simulink library "MotoLibrary"  (R2019b)
settings: Solver=VariableStepAuto  StartTime=0.0  StopTime=10.0  RelTol=1e-3
undefined symbols (not defined in the file or in its folder): Percentage
libraries: arduinolib x9, simulink x2, $bdroot x2
settings Model: Creator=JB  LastModifiedBy=JB

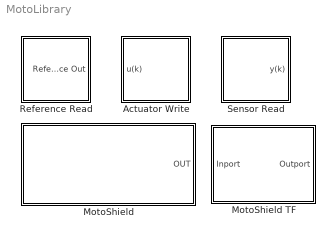
== system MotoLibrary ==
  Actuator Write : Subsystem  mask{inputType=Percentage (%), dir=Clockwise}
      mask prompts: inputType "Selected Input Type:"; dir "Spin Direction:"
      mask init:
      | if dir == 1
      |     direction = 1
      | else
      |     direction = 0
      | end
      mask TypeOptions inputType: Percentage (%) | Voltage (V) | PWM (8-bit)
      mask Callback inputType:
      | obj = get_param(gcb,'MaskObject');
      | txt = obj.getDialogControl('text');
      | input = get_param(gcb,'inputType');
      | if strcmp(input, 'Percentage (%)')
      |     txt.Prompt = 'Expected input value ranges between 0 - 100 %';
      | end
      | if strcmp(input, 'Voltage (V)')
      |     txt.Prompt = 'Expected input value ranges between 0 - 5 V';
      | end
      | if strcmp(input, 'PWM (8-bit)')
      |     txt.Prompt = 'Expected input value ranges between 0 - 255';
      | end
      mask TypeOptions dir: Clockwise | Counter-clockwise
      mask DialogControl DescGroupVar Prompt: MotoShield Actuator
      mask DialogControl DescTextVar Prompt: This block writes PWM signal to motor in MotoShield device. Expected input value varies based on the Selected Input Type.
      mask DialogControl text Prompt: Expected input value ranges between 0 - 100 %
      mask Display: image('assets\MotoShield_Motor.svg');
  MotoShield : Subsystem  mask{inputType=Internal Reference, direction=Clockwise, calibration=Perform calibration, manualLower=1010, manualUpper=2120, Ts=0.1}
      mask prompts: inputType "Form of input:"; calibration "Calibration values:"; manualLower "Minimal value:"; manualUpper "Maximal value:"; Ts "Sampling time (s):"
      mask init:
      | set_param(gcb, 'MaskSelfModifiable', 'on');
      | if inputType == 1
      |     if getSimulinkBlockHandle([gcb '/Inport']) == -1
      |         delete_line(gcb,'Reference Read/1','Saturation/1');
      |         add_block('built-in/Inport',[gcb '/Inport']);
      |         add_line(gcb,'Inport/1','Saturation/1');
      |     end
      | elseif inputType == 2
      |     if getSimulinkBlockHandle([gcb '/Inport']) > 0
      |         delete_line(gcb,'Inport/1','Saturation/1');
      |         delete_block([gcb '/Inport']);
      |         add_line(gcb,'Reference Read/1','Saturation/1');
      |     end
      | end
      mask TypeOptions inputType: External Reference | Internal Reference
      mask TypeOptions direction: Clockwise | Counterclockwise
      mask TypeOptions calibration: Perform calibration | Use default values | Set values manually
      mask Callback calibration:
      | currentBlock = gcb
      | in = get_param(currentBlock,'calibration');
      | menu = Simulink.Mask.get(currentBlock);
      | txt = menu.getDialogControl('calText');
      | lower = menu.getParameter('manualLower');
      | upper = menu.getParameter('manualUpper');
      | if strcmp(in,'Perform calibration')
      | lower.Enabled='off';
      | lower.Visible='off';
      | upper.Enabled='off';
      | upper.Visible='off';
      | txt.Visible='off';
      | elseif strcmp(in,'Use default values')
      | lower.Enabled='off';
      | lower.Visible='on';
      | upper.Enabled='off';
      | upper.Visible='on';
      | set_param(gcb,'manualLower',num2str(800));
      | set_param(gcb,'manualUpper',num2str(2050));
      | elseif strcmp(in,'Set values manually')
      | lower.Enabled='on';
      | lower.Visible='on';
      | upper.Enabled='on';
      | upper.Visible='on';
      | txt.Visible='on';
      | end
      mask DialogControl DescGroupVar Prompt: MotoShield
      mask DialogControl DescTextVar Prompt: This blocks writes actuator value and measures the angular velocity of the Motor. The reference value can be chosen either as an external signal or internal potentiometers value.  Since the output signal is expressed in percentages, calibration values have to be either specified or aquired via calibration. It is recommended to perform a calibration for accurate percentage formatting.
      mask DialogControl Control2 Prompt: Notice: Calibration is applicable only for unladen state.
      mask DialogControl calText Prompt: Calibration values ought to be entered as angular velocity in number of impulses per sample.
      mask Display: image('assets\MotoShield.svg');
  MotoShield TF : Subsystem  mask{inputType=Percentage (%), outputType=Rotations per minute (RPM), maxValue=0, minValue=0}
      mask prompts: inputType "Input value type:"; outputType "Output value type:"; maxValue "Calibration maximum value:"; minValue "Calibration minimum value:"
      mask TypeOptions inputType: Percentage (%) | RMS Voltage (V)
      mask TypeOptions outputType: Rotations per minute (RPM) | Radians per second (rad/s) | Percentage (%)
      mask Callback outputType:
      | CurrentBlock = gcb;
      | cal = get_param(CurrentBlock,'outputType');
      | menu = Simulink.Mask.get(CurrentBlock);
      | txt = menu.getDialogControl('calText');
      | min = menu.getParameter('minValue');
      | max = menu.getParameter('maxValue');
      | if strcmp(cal,'Percentage (%)')
      | min.Enabled='on';
      | min.Visible='on';
      | max.Enabled='on';
      | max.Visible='on';
      | txt.Visible='on';
      | set_param(gcb,'minValue',num2str(488));
      | set_param(gcb,'maxValue',num2str(976));
      | else
      | min.Enabled='off';
      | min.Visible='off';
      | max.Enabled='off';
      | max.Visible='off';
      | txt.Visible='off';
      | end
      mask DialogControl DescGroupVar Prompt: OptoShield TF
      mask DialogControl DescTextVar Prompt: The block represents the simplified second-order continuous transfer function of the MotoShield device.   Both input and output are availible in several value types. If output type selected is Percentage (%), calibration values are required. The calibration values have to be stated in radians per second.
      mask DialogControl Container2 Prompt: Parameters
      mask DialogControl calText Prompt: Calibration values are supposed to represent output range of the Motor in Radian per second (rad/s).
      mask Display: image('assets\MotoShield_TF.svg');
  Reference Read : Subsystem  mask{radio=Percentage (%), Ts=0.1}
      mask prompts: radio "Readout Type"; Ts "Sample time (s):"
      mask init:
      | if radio==1 
      | gainValue = (100/1023);       
      | end
      | if radio==2
      | gainValue = (5/1023);
      | end
      | if radio==3
      | gainValue = 1;             
      | end
      mask TypeOptions radio: Percentage (%) | Voltage (V) | Analog value (10-bit ADC)
      mask DialogControl DescGroupVar Prompt: MotoShield Potentiometer
      mask DialogControl DescTextVar Prompt: This blocks reads potentiometer wiper value on the MotoShield device. Multiple output value types availible.
      mask Display: image('assets\Potentiometer.svg');
  Sensor Read : Subsystem  mask{outputType=Percentage (%), calibrationValues=Use default values, minValue=800, maxValue=2060, Ts=0.1}
      mask prompts: outputType "Selected Output Type:"; calibrationValues "Calibration Values:"; minValue "Minimal Value:"; maxValue "Maximal Value:"; Ts "Sample time (s):"
      mask TypeOptions outputType: Percentage (%) | Rotation per minute (RPM) | Radian per second (rad/s)
      mask Callback outputType:
      | CurrentBlock = gcb;
      | out = get_param(CurrentBlock,'outputType');
      | menu = Simulink.Mask.get(CurrentBlock);
      | txt = menu.getDialogControl('calText');
      | calopt = menu.getParameter('calibrationValues');
      | min = menu.getParameter('minValue');
      | max = menu.getParameter('maxValue');
      | if strcmp(out,'Percentage (%)')
      | calopt.Enabled='on';
      | calopt.Visible='on';
      | txt.Visible='on';
      | else
      | calopt.Enabled='off';
      | calopt.Visible='off';
      | min.Visible = 'off'
      | max.Visible = 'off'
      | txt.Visible='off';
      | end
      mask TypeOptions calibrationValues: Set values manually | Use default values
      mask Callback calibrationValues:
      | CurrentBlock = gcbh;
      | cal = get_param(CurrentBlock,'calibrationValues');
      | menu = Simulink.Mask.get(CurrentBlock);
      | min = menu.getParameter('minValue');
      | max = menu.getParameter('maxValue');
      | if strcmp(cal,'Set values manually')
      | min.Enabled='on';
      | min.Visible='on';
      | max.Enabled='on';
      | max.Visible='on';
      | elseif strcmp(cal,'Use default values')
      | set_param(gcb,'minValue',num2str(800));
      | set_param(gcb,'maxValue',num2str(2060));
      | min.Enabled='off';
      | min.Visible='on';
      | max.Enabled='off';
      | max.Visible='on';
      | end
      mask DialogControl DescGroupVar Prompt: Hall Sensor
      mask DialogControl DescTextVar Prompt: This block outputs the angular velocity of the Motor. Multiple output value types available.
      mask DialogControl calText Prompt: Calibration values ought to be entered as angular velocity in number of impulses per sample.
      mask Display: image('assets\MotoShield_Sensor.svg');

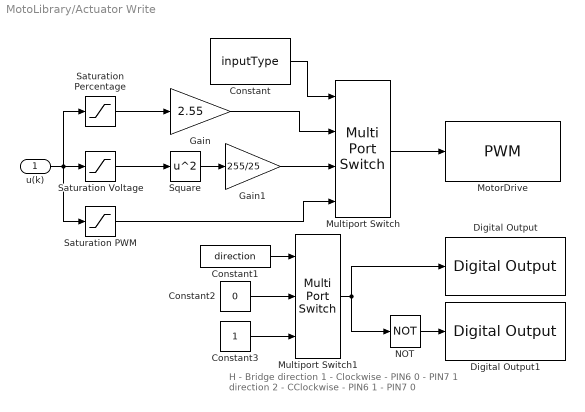
== system MotoLibrary/Actuator Write ==
  note: H - Bridge
      | direction 1 - Clockwise - PIN6 0 - PIN7 1
      | direction 2 - CClockwise - PIN6 1 - PIN7 0
  u(k) : Inport
  Constant : Constant  Value=inputType
  Constant1 : Constant  Value=direction
  Constant2 : Constant  Value=0
  Constant3 : Constant
  Digital Output : arduinolib/Digital Output  pinNumber=6  blockPlatform=arduino
  Digital Output1 : arduinolib/Digital Output  pinNumber=7  blockPlatform=arduino
  Gain : Gain  Gain=2.55
  Gain1 : Gain  Gain=255/25
  MotorDrive : arduinolib/PWM  pinNumber=5  EnableInputFrequency=off  InitialFrequency=2000  InitialDutyCycle=0  NotificationType=None  blockPlatform=arduino
  Multiport Switch : MultiPortSwitch
  Multiport Switch1 : MultiPortSwitch  Inputs=2
  NOT : Logic  Operator=NOT  IconShape=distinctive  AllPortsSameDT=off  OutDataTypeStr=boolean
  Saturation PWM : Saturate  UpperLimit=255  LowerLimit=0
  Saturation Percentage : Saturate  UpperLimit=100  LowerLimit=0
  Saturation Voltage : Saturate  UpperLimit=5  LowerLimit=0
  Square : Math  Operator=square  SignedPower=off  SaturateOnIntegerOverflow=on
  wires:
  Saturation Percentage/1 -> Gain/1
  Constant/1 -> Multiport Switch/1
  Gain/1 -> Multiport Switch/2
  Saturation Voltage/1 -> Square/1
  Square/1 -> Gain1/1
  Gain1/1 -> Multiport Switch/3
  Multiport Switch/1 -> MotorDrive/1
  u(k)/1 -> Saturation PWM/1, Saturation Percentage/1, Saturation Voltage/1
  Saturation PWM/1 -> Multiport Switch/4
  Constant1/1 -> Multiport Switch1/1
  Constant2/1 -> Multiport Switch1/2
  Constant3/1 -> Multiport Switch1/3
  Multiport Switch1/1 -> Digital Output/1, NOT/1
  NOT/1 -> Digital Output1/1

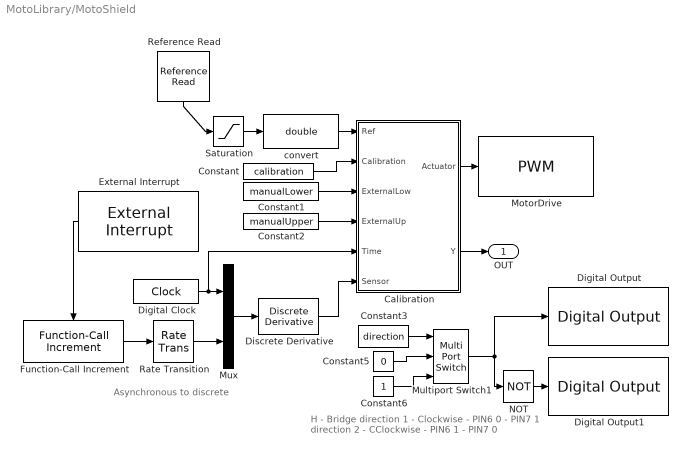
== system MotoLibrary/MotoShield ==
  note: Asynchronous to discrete
  note: H - Bridge
      | direction 1 - Clockwise - PIN6 0 - PIN7 1
      | direction 2 - CClockwise - PIN6 1 - PIN7 0
  Calibration : MATLAB Function  TreatAsAtomicUnit=on
  Constant : Constant  Value=calibration
  Constant1 : Constant  Value=manualLower
  Constant2 : Constant  Value=manualUpper
  Constant3 : Constant  Value=direction
  Constant5 : Constant  Value=0
  Constant6 : Constant
  Digital Clock : DigitalClock  SampleTime=Ts
  Digital Output : arduinolib/Digital Output  pinNumber=6  blockPlatform=arduino
  Digital Output1 : arduinolib/Digital Output  pinNumber=7  blockPlatform=arduino
  Discrete Derivative : simulink/Quick Insert/Discrete/Discrete Derivative  gainval=1.0  ICPrevScaledInput=0.0  OutMin=[]  OutMax=[]  OutDataType=fixdt(1, 16)  OutScaling=2^-10  DoSatur=off
      settings: SourceProductName=Simulink  SourceProductBaseCode=SL
  External Interrupt : arduinolib/External Interrupt  Pin=3  PullUp=off  Mode=CHANGE  InterruptSimulationInput=off
      settings: SourceProductName=Simulink Support Package for Arduino Hardware  SourceProductBaseCode=ARDUINO
  Function-Call Increment : $bdroot/Sensor Read/Function-Call Increment  SystemSampleTime=-1  Latency=0  AutoFrameSizeCalculation=off
  MotorDrive : arduinolib/PWM  pinNumber=5  EnableInputFrequency=off  InitialFrequency=2000  InitialDutyCycle=0  NotificationType=None  blockPlatform=arduino
  Multiport Switch1 : MultiPortSwitch  Inputs=2
  Mux : Mux  Inputs=2
  NOT : Logic  Operator=NOT  IconShape=distinctive  AllPortsSameDT=off  OutDataTypeStr=boolean
  Rate Transition : RateTransition  Deterministic=off  OutPortSampleTimeOpt=Inherit  OutPortSampleTime=0.01
  Reference Read : $bdroot/Reference Read  radio=Percentage (%)  Ts=Ts
  Saturation : Saturate  UpperLimit=100  LowerLimit=0
  convert : DataTypeConversion  OutDataTypeStr=double
  OUT : Outport
  wires:
  Multiport Switch1/1 -> NOT/1, Digital Output/1
  NOT/1 -> Digital Output1/1
  Constant6/1 -> Multiport Switch1/3
  Constant5/1 -> Multiport Switch1/2
  External Interrupt/1 -> Function-Call Increment/Trigger
  Digital Clock/1 -> Calibration/5(Time), Mux/1
  Rate Transition/1 -> Mux/2
  Mux/1 -> Discrete Derivative/1
  Function-Call Increment/1 -> Rate Transition/1
  Constant3/1 -> Multiport Switch1/1
  Calibration/1(Actuator) -> MotorDrive/1
  Constant/1 -> Calibration/2(Calibration)
  Constant1/1 -> Calibration/3(ExternalLow)
  Constant2/1 -> Calibration/4(ExternalUp)
  Discrete Derivative/1 -> Calibration/6(Sensor)
  convert/1 -> Calibration/1(Ref)
  Saturation/1 -> convert/1
  Reference Read/1 -> Saturation/1
  Calibration/2(Y) -> OUT/1

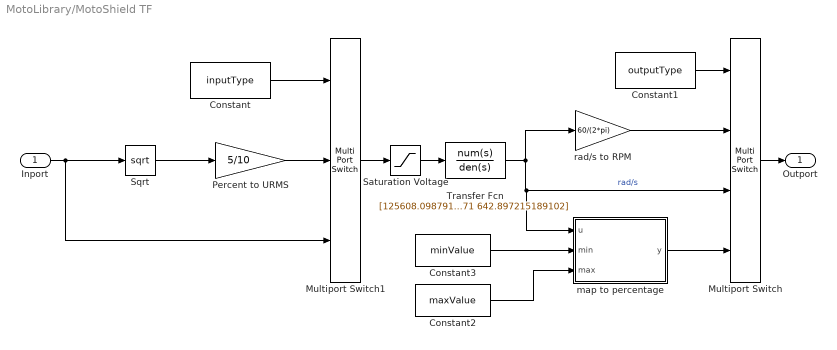
== system MotoLibrary/MotoShield TF ==
  Inport : Inport
  Constant : Constant  Value=inputType
  Constant1 : Constant  Value=outputType
  Constant2 : Constant  Value=maxValue
  Constant3 : Constant  Value=minValue
  Multiport Switch : MultiPortSwitch
  Multiport Switch1 : MultiPortSwitch  Inputs=2
  Percent to URMS : Gain  Gain=5/10
  Saturation Voltage : Saturate  UpperLimit=5  LowerLimit=0
  Sqrt : Sqrt  SaturateOnIntegerOverflow=on
  Transfer Fcn : TransferFcn  Numerator=[125608.098791341]  Denominator=[1 84.2769333261671 642.897215189102]  ContinuousStateAttributes='velocity'
  map to percentage : MATLAB Function  TreatAsAtomicUnit=on
  rad/s to RPM : Gain  Gain=60/(2*pi)
  Outport : Outport
  wires:
  Multiport Switch/1 -> Outport/1
  Constant1/1 -> Multiport Switch/1
  Constant/1 -> Multiport Switch1/1
  Inport/1 -> Multiport Switch1/3, Sqrt/1
  Multiport Switch1/1 -> Saturation Voltage/1
  Transfer Fcn/1 -> map to percentage/1(u), Multiport Switch/3, rad/s to RPM/1  "rad/s"
  rad/s to RPM/1 -> Multiport Switch/2
  map to percentage/1(y) -> Multiport Switch/4
  Sqrt/1 -> Percent to URMS/1
  Percent to URMS/1 -> Multiport Switch1/2
  Saturation Voltage/1 -> Transfer Fcn/1
  Constant3/1 -> map to percentage/2(min)
  Constant2/1 -> map to percentage/3(max)

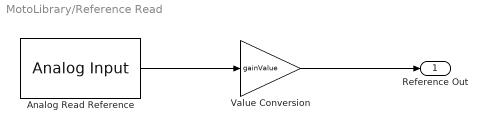
== system MotoLibrary/Reference Read ==
  Analog Read Reference : arduinolib/Analog Input  pinNumber=4  ReadResultsOnly=off  ConversionTriggerSource=Software  ExternalTriggerType=uint32(0)  OutputDataType=uint16  EnableConversionCompleteNotify=off  EnableOuputStatus=off  SampleTime=Ts  blockPlatform=arduino
  Value Conversion : Gain  Gain=gainValue
  Reference Out : Outport
  wires:
  Analog Read Reference/1 -> Value Conversion/1
  Value Conversion/1 -> Reference Out/1

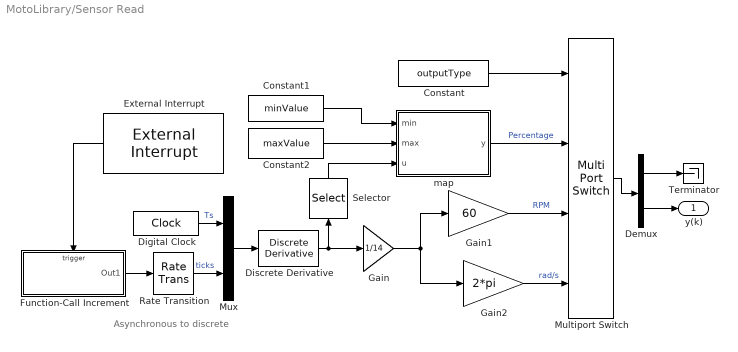
== system MotoLibrary/Sensor Read ==
  note: Asynchronous to discrete
  Constant : Constant  Value=outputType
  Constant1 : Constant  Value=minValue
  Constant2 : Constant  Value=maxValue
  Demux : Demux  Outputs=2
  Digital Clock : DigitalClock  SampleTime=Ts
  Discrete Derivative : simulink/Quick Insert/Discrete/Discrete Derivative  gainval=1.0  ICPrevScaledInput=0.0  OutMin=[]  OutMax=[]  OutDataType=fixdt(1, 16)  OutScaling=2^-10  DoSatur=off
      settings: SourceProductName=Simulink  SourceProductBaseCode=SL
  External Interrupt : arduinolib/External Interrupt  Pin=3  PullUp=off  Mode=CHANGE  InterruptSimulationInput=off
      settings: SourceProductName=Simulink Support Package for Arduino Hardware  SourceProductBaseCode=ARDUINO
  Function-Call Increment : Subsystem  TreatAsAtomicUnit=on
  Gain : Gain  Gain=1/14
  Gain1 : Gain  Gain=60
  Gain2 : Gain  Gain=2*pi
  Multiport Switch : MultiPortSwitch
  Mux : Mux  Inputs=2
  Rate Transition : RateTransition  Deterministic=off  OutPortSampleTimeOpt=Inherit  OutPortSampleTime=0.01
  Selector : Selector  InputPortWidth=2  IndexOptions=Index vector (dialog)  Indices=2  OutputSizes=1
  Terminator : Terminator
  map : MATLAB Function  TreatAsAtomicUnit=on
  y(k) : Outport
  wires:
  External Interrupt/1 -> Function-Call Increment/Trigger
  Function-Call Increment/1(Out1) -> Rate Transition/1
  Digital Clock/1 -> Mux/1  "Ts"
  Mux/1 -> Discrete Derivative/1
  Rate Transition/1 -> Mux/2  "ticks"
  Discrete Derivative/1 -> Selector/1, Gain/1
  Gain/1 -> Gain2/1, Gain1/1
  Gain2/1 -> Multiport Switch/4  "rad/s"
  Gain1/1 -> Multiport Switch/3  "RPM"
  Constant/1 -> Multiport Switch/1
  map/1(y) -> Multiport Switch/2  "Percentage"
  Constant1/1 -> map/1(min)
  Constant2/1 -> map/2(max)
  Selector/1 -> map/3(u)
  Multiport Switch/1 -> Demux/1
  Demux/2 -> y(k)/1
  Demux/1 -> Terminator/1

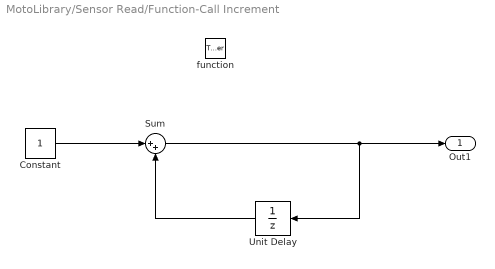
== system MotoLibrary/Sensor Read/Function-Call Increment ==
  function : TriggerPort  TriggerType=function-call  VariantControl=Variant
  Constant : Constant
  Sum : Sum  Inputs=|++
  Unit Delay : UnitDelay  SampleTime=-1  HasFrameUpgradeWarning=on
  Out1 : Outport  VectorParamsAs1DForOutWhenUnconnected=off
  wires:
  Sum/1 -> Unit Delay/1, Out1/1
  Constant/1 -> Sum/1
  Unit Delay/1 -> Sum/2

== matlab function MotoLibrary/MotoShield TF/map to percentage ==
  data: u input; min input; max input; y output
%     Matlab function for Sensor Read block.
%
%     This code is part of the AutomationShield hardware and software
%     ecosystem. Visit http://www.automationshield.com for more
%     details. This code is licensed under a Creative Commons
%     Attribution-NonCommercial 4.0 International License.
%
%     Created by: Jan Boldocky
%     Last update: 19.05.2020
function y = fcn(u,min,max)
   y = constrain(map(u, min, max, 0, 100), 0, 100);
end

== matlab function MotoLibrary/Sensor Read/map ==
  data: min input; max input; u input; y output
%     Matlab function for Sensor Read block.
%
%     This code is part of the AutomationShield hardware and software
%     ecosystem. Visit http://www.automationshield.com for more
%     details. This code is licensed under a Creative Commons
%     Attribution-NonCommercial 4.0 International License.
%
%     Created by: Jan Boldocky
%     Last update: 19.05.2020
function y = fcn(min,max,u)
   y = constrain(map(u, min, max, 0, 100), 0, 100);
end

== matlab function MotoLibrary/MotoShield/Calibration ==
  data: Ref input; Calibration input; ExternalLow input; ExternalUp input; Time input; Sensor input; Actuator output; Y output
%     Matlab function for MotoShield block functionality/calibration.
%
%     This code is part of the AutomationShield hardware and software
%     ecosystem. Visit http://www.automationshield.com for more
%     details. This code is licensed under a Creative Commons
%     Attribution-NonCommercial 4.0 International License.
%
%     Created by: Jan Boldocky
%     Last update: 19.05.2020
function [Actuator, Y] = fcn(Ref,Calibration,ExternalLow,ExternalUp,Time,Sensor) %_inputs/outputs
persistent i t timeMem Upper Lower WasCalibrated; %_persistent variables

if isempty(Upper) %_first run condition
    Lower = 0; %_mapping values
    Upper = 0;
    i = 40; %_Presumed Min PWM 8-bit
    t=0; %_Sampling variable
    WasCalibrated = 0; %_true/false variable
end
Actuator = 0; %_Initial value
if (Calibration == 1) && (WasCalibrated == 0) %_if calibration selected and hasnt been performed yet
    if Time < 2.1   %_Until 2.1s
        Actuator = 255; %_spin motor max PWM
        if Time >= 2  %_at 2 sec
            Upper = Sensor(2); %_sense maxRPM 
        end
    end
    if (Time >= 3) %_if 3 seconds has passed
        Actuator = i; %_value i to actuator
        if Time >= 3+t %_if next Sample
            t = t + 0.1; %_increment Sample
            i = i + 1;    %_increment Actuator
        end
        if Sensor(2) > 400 %_motion condition
            i = i - 1; %_if motor started spinning, dont increment Actuator value
            if isempty(timeMem)%_use timeMem only once
                timeMem = Time; %_memorise time
            end
            if Time >= timeMem + 1.5 %_waiting to stabilize @ minimal Value
                Lower = Sensor(2); %_sense minRPM
                WasCalibrated = 1; %_END OF CALIBRATION
            end
        end
    end
end
if (Calibration ~= 1) && (Upper == 0)%_if calibration was NOT selected && ONLY ONCE
Upper = ExternalUp; %_mapping variables are assigned Manually entered Value
Lower = ExternalLow;
WasCalibrated = 1;
end
if(WasCalibrated == 1) %_actuator Value after calibration
    Actuator = Ref*2.55; 
end
Y = constrain(map(Sensor(2),Lower,Upper,0,100),0,100);%_OUTPUT value #constrained mapped#
